simulink model "bench"  (R2025b)
settings: Solver=ode4  StartTime=0.0  StopTime=inf  FixedStep=Ts_gcs  RelTol=1e-3
InitFcn:
  | bench_init_fcn(mocap);
undefined symbols (not defined in the file): mocap, Ts_gcs
libraries: instrumentseriallib x2, sldrtlib x1
settings Model: DataDictionary=project.sldd  SimulationMode=accelerator  Creator=Nick  LastModifiedBy=Rakete
settings SolverCC: AutoInsertRateTranBlk=on

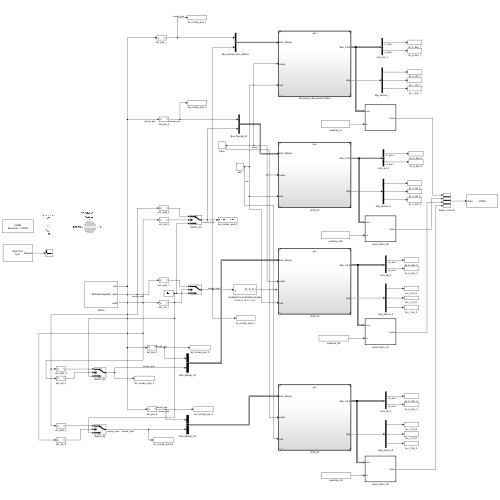
[thumbnail: Simulink's stored preview of the top-level diagram]
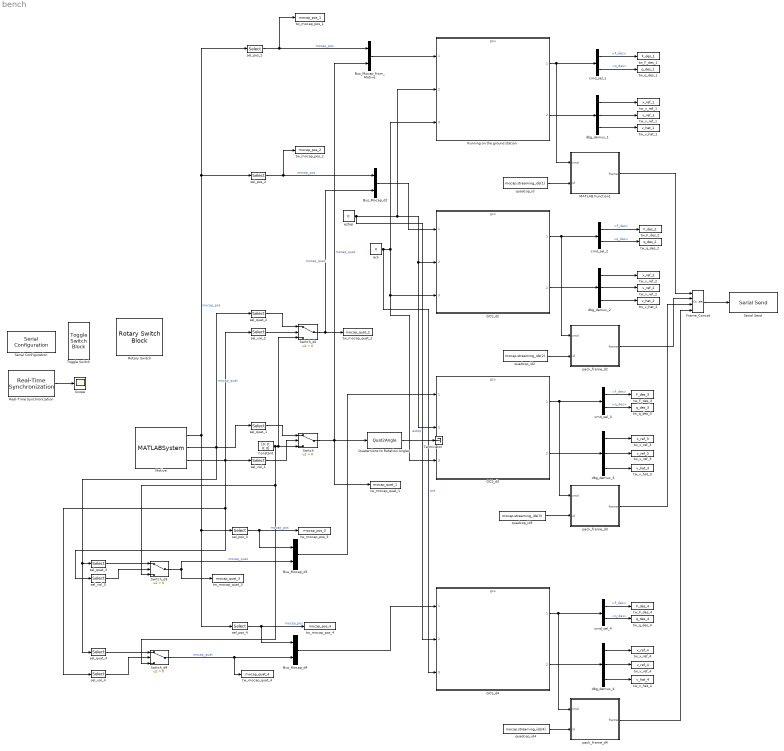
== system bench ==
  Bus_Mocap_d2 : BusCreator  Inputs=2  OutDataTypeStr=Bus: Bus_Mocap
  Bus_Mocap_d3 : BusCreator  Inputs=2  OutDataTypeStr=Bus: Bus_Mocap
  Bus_Mocap_d4 : BusCreator  Inputs=2  OutDataTypeStr=Bus: Bus_Mocap
  Bus_Mocap_from_Motive : BusCreator  Inputs=2  OutDataTypeStr=Bus: Bus_Mocap
  Constant : Constant  Value=[0; 0; 0; 0]
  Frame_Concat : Concatenate  NumInputs=4
  GCS_d2 : ModelReference  ModelNameDialog=gcu.slx  UsingDefaultArgumentValue=0,0,0  SimulationMode=Normal  ModelReferenceVersion=1.334
  GCS_d3 : ModelReference  ModelNameDialog=gcu.slx  UsingDefaultArgumentValue=0,0,0  SimulationMode=Normal  ModelReferenceVersion=1.334
  GCS_d4 : ModelReference  ModelNameDialog=gcu.slx  UsingDefaultArgumentValue=0,0,0  SimulationMode=Normal  ModelReferenceVersion=1.334
  MATLAB Function1 : MATLAB Function  TreatAsAtomicUnit=on
  Motive : MATLABSystem  System=MotiveMocapMulti  HostIP=mocap.host_ip  ClientIP=mocap.client_ip  StreamingIDs=mocap.streaming_ids  SampleTimeSec=Ts_gcs  Verbose=on
      mask Type: MotiveMocapMulti
  Quaternions to Rotation Angles : Quat2Angle
      settings: AttributesFormatString=Rotation Order: %<rotationOrder>
  Real-Time Synchronization : sldrtlib/Real-Time Synchronization  SampleTime=Ts_gcs  MaxMissedTicks=inf  ShowMissedTicks=on  YieldWhenWaiting=off
  Rotary Switch : RotarySwitchBlock
  Running on the ground station : ModelReference  ModelNameDialog=gcu.slx  UsingDefaultArgumentValue=0,0,0  SimulationMode=Normal  ModelReferenceVersion=1.334
  Scope : Scope
      settings: ActiveDisplayYMinimum=-1  ActiveDisplayYMaximum=1
  Serial Configuration : instrumentseriallib/Serial Configuration  Priority=-200000  PortSel=COM4  Port=COM4  ComPort=COM4  BaudRate=115200  DataBits=8  Parity=none  StopBits=1  ByteOrder=little-endian  FlowControl=none  Timeout=10  SimulateUsing=Interpreted execution  BlockInModel=on  aMode=1
      settings: LibrarySourceBlock=c2000lib/Host Communication/Serial Configuration
  Serial Send : instrumentseriallib/Serial Send  Priority=1  PortSel=COM4  Port=COM4  ComPort=COM4  Header=[]  Terminator=<none>  CustomTerminator=[]  EnableBlockingMode=on  SimulateUsing=Interpreted execution  BlockInModel=on  aMode=1
      settings: LibrarySourceBlock=c2000lib/Host Communication/Serial Send
  Switch : Switch  Criteria=u2 > Threshold  SaturateOnIntegerOverflow=off  InputSameDT=off
  Switch_d2 : Switch  Criteria=u2 > Threshold  SaturateOnIntegerOverflow=off  InputSameDT=off
  Switch_d3 : Switch  Criteria=u2 > Threshold  SaturateOnIntegerOverflow=off  InputSameDT=off
  Switch_d4 : Switch  Criteria=u2 > Threshold  SaturateOnIntegerOverflow=off  InputSameDT=off
  Terminator : Terminator
  Toggle Switch : ToggleSwitchBlock
  ack : Constant  Value=0  OutDataTypeStr=boolean
  cmd_sel_{1..4} (4 alike) : BusSelector  OutputSignals=F_des,q_des
  dbg_demux_{1..4} (4 alike) : Demux  Outputs=[3 3 3]
  estop : Constant  Value=0  OutDataTypeStr=uint8
  pack_frame_d2 : MATLAB Function  TreatAsAtomicUnit=on
  pack_frame_d3 : MATLAB Function  TreatAsAtomicUnit=on
  pack_frame_d4 : MATLAB Function  TreatAsAtomicUnit=on
  quadcop_id : Constant  Value=mocap.streaming_ids(1)  OutDataTypeStr=uint8
  quadcop_id2 : Constant  Value=mocap.streaming_ids(2)  OutDataTypeStr=uint8
  quadcop_id3 : Constant  Value=mocap.streaming_ids(3)  OutDataTypeStr=uint8
  quadcop_id4 : Constant  Value=mocap.streaming_ids(4)  OutDataTypeStr=uint8
  sel_pos_1 : Selector  NumberOfDimensions=2  IndexOptions=Select all,Index vector (dialog)  Indices=1,1  OutputSizes=1
  sel_pos_2 : Selector  NumberOfDimensions=2  IndexOptions=Select all,Index vector (dialog)  Indices=1,2  OutputSizes=1
  sel_pos_3 : Selector  NumberOfDimensions=2  IndexOptions=Select all,Index vector (dialog)  Indices=1,3  OutputSizes=1
  sel_pos_4 : Selector  NumberOfDimensions=2  IndexOptions=Select all,Index vector (dialog)  Indices=1,4  OutputSizes=1
  sel_quat_1 : Selector  NumberOfDimensions=2  IndexOptions=Select all,Index vector (dialog)  Indices=1,1  OutputSizes=1
  sel_quat_2 : Selector  NumberOfDimensions=2  IndexOptions=Select all,Index vector (dialog)  Indices=1,2  OutputSizes=1
  sel_quat_3 : Selector  NumberOfDimensions=2  IndexOptions=Select all,Index vector (dialog)  Indices=1,3  OutputSizes=1
  sel_quat_4 : Selector  NumberOfDimensions=2  IndexOptions=Select all,Index vector (dialog)  Indices=1,4  OutputSizes=1
  sel_val_1 : Selector  IndexOptions=Index vector (dialog)  Indices=1  OutputSizes=1
  sel_val_2 : Selector  IndexOptions=Index vector (dialog)  Indices=2  OutputSizes=1
  sel_val_3 : Selector  IndexOptions=Index vector (dialog)  Indices=3  OutputSizes=1
  sel_val_4 : Selector  IndexOptions=Index vector (dialog)  Indices=4  OutputSizes=1
  tw_F_des_1 : ToWorkspace  VariableName=F_des_1  SaveFormat=Timeseries  SampleTime=Ts_gcs
  tw_F_des_2 : ToWorkspace  VariableName=F_des_2  SaveFormat=Timeseries  SampleTime=Ts_gcs
  tw_F_des_3 : ToWorkspace  VariableName=F_des_3  SaveFormat=Timeseries  SampleTime=Ts_gcs
  tw_F_des_4 : ToWorkspace  VariableName=F_des_4  SaveFormat=Timeseries  SampleTime=Ts_gcs
  tw_mocap_pos_1 : ToWorkspace  VariableName=mocap_pos_1  SaveFormat=Timeseries  SampleTime=Ts_gcs
  tw_mocap_pos_2 : ToWorkspace  VariableName=mocap_pos_2  SaveFormat=Timeseries  SampleTime=Ts_gcs
  tw_mocap_pos_3 : ToWorkspace  VariableName=mocap_pos_3  SaveFormat=Timeseries  SampleTime=Ts_gcs
  tw_mocap_pos_4 : ToWorkspace  VariableName=mocap_pos_4  SaveFormat=Timeseries  SampleTime=Ts_gcs
  tw_mocap_quat_1 : ToWorkspace  VariableName=mocap_quat_1  SaveFormat=Timeseries  SampleTime=Ts_gcs
  tw_mocap_quat_2 : ToWorkspace  VariableName=mocap_quat_2  SaveFormat=Timeseries  SampleTime=Ts_gcs
  tw_mocap_quat_3 : ToWorkspace  VariableName=mocap_quat_3  SaveFormat=Timeseries  SampleTime=Ts_gcs
  tw_mocap_quat_4 : ToWorkspace  VariableName=mocap_quat_4  SaveFormat=Timeseries  SampleTime=Ts_gcs
  tw_q_des_1 : ToWorkspace  VariableName=q_des_1  SaveFormat=Timeseries  SampleTime=Ts_gcs
  tw_q_des_2 : ToWorkspace  VariableName=q_des_2  SaveFormat=Timeseries  SampleTime=Ts_gcs
  tw_q_des_3 : ToWorkspace  VariableName=q_des_3  SaveFormat=Timeseries  SampleTime=Ts_gcs
  tw_q_des_4 : ToWorkspace  VariableName=q_des_4  SaveFormat=Timeseries  SampleTime=Ts_gcs
  tw_v_hat_1 : ToWorkspace  VariableName=v_hat_1  SaveFormat=Timeseries  SampleTime=Ts_gcs
  tw_v_hat_2 : ToWorkspace  VariableName=v_hat_2  SaveFormat=Timeseries  SampleTime=Ts_gcs
  tw_v_hat_3 : ToWorkspace  VariableName=v_hat_3  SaveFormat=Timeseries  SampleTime=Ts_gcs
  tw_v_hat_4 : ToWorkspace  VariableName=v_hat_4  SaveFormat=Timeseries  SampleTime=Ts_gcs
  tw_v_ref_1 : ToWorkspace  VariableName=v_ref_1  SaveFormat=Timeseries  SampleTime=Ts_gcs
  tw_v_ref_2 : ToWorkspace  VariableName=v_ref_2  SaveFormat=Timeseries  SampleTime=Ts_gcs
  tw_v_ref_3 : ToWorkspace  VariableName=v_ref_3  SaveFormat=Timeseries  SampleTime=Ts_gcs
  tw_v_ref_4 : ToWorkspace  VariableName=v_ref_4  SaveFormat=Timeseries  SampleTime=Ts_gcs
  tw_x_ref_1 : ToWorkspace  VariableName=x_ref_1  SaveFormat=Timeseries  SampleTime=Ts_gcs
  tw_x_ref_2 : ToWorkspace  VariableName=x_ref_2  SaveFormat=Timeseries  SampleTime=Ts_gcs
  tw_x_ref_3 : ToWorkspace  VariableName=x_ref_3  SaveFormat=Timeseries  SampleTime=Ts_gcs
  tw_x_ref_4 : ToWorkspace  VariableName=x_ref_4  SaveFormat=Timeseries  SampleTime=Ts_gcs
  wires:
  sel_val_1/1 -> Switch/2
  Motive/3 -> sel_val_3/1, sel_val_4/1, sel_val_1/1, sel_val_2/1
  Motive/1 -> sel_pos_3/1, sel_pos_4/1, sel_pos_2/1, sel_pos_1/1  "mocap_pos"
  Motive/2 -> sel_quat_3/1, sel_quat_4/1, sel_quat_1/1, sel_quat_2/1  "mocap_quat"
  quadcop_id2/1 -> pack_frame_d2/2(id)
  Real-Time Synchronization/1 -> Scope/1
  dbg_demux_2/1 -> tw_x_ref_2/1
  sel_pos_1/1 -> tw_mocap_pos_1/1, Bus_Mocap_from_Motive/1  "mocap_pos"
  sel_val_2/1 -> Switch_d2/2
  Switch_d2/1 -> tw_mocap_quat_2/1, Bus_Mocap_d2/2  "mocap_quat"
  sel_quat_1/1 -> Switch/1
  sel_quat_2/1 -> Switch_d2/1
  sel_pos_2/1 -> Bus_Mocap_d2/1, tw_mocap_pos_2/1  "mocap_pos"
  Constant/1 -> Switch_d3/3, Switch_d4/3, Switch/3, Switch_d2/3
  GCS_d2/1 -> pack_frame_d2/1(cmd), cmd_sel_2/1
  Switch/1 -> Quaternions to Rotation Angles/1, tw_mocap_quat_1/1, Bus_Mocap_from_Motive/2  "mocap_quat"
  Running on the ground station/2 -> dbg_demux_1/1
  Bus_Mocap_from_Motive/1 -> Running on the ground station/1
  MATLAB Function1/1(frame) -> Frame_Concat/1
  Bus_Mocap_d2/1 -> GCS_d2/1
  dbg_demux_1/2 -> tw_v_ref_1/1
  estop/1 -> GCS_d3/2, GCS_d2/2, Running on the ground station/2, GCS_d4/2  "estop"
  ack/1 -> GCS_d3/3, GCS_d2/3, Running on the ground station/3, GCS_d4/3  "ack"
  dbg_demux_1/3 -> tw_v_hat_1/1
  Running on the ground station/1 -> MATLAB Function1/1(cmd), cmd_sel_1/1
  Quaternions to Rotation Angles/1 -> Terminator/1
  GCS_d2/2 -> dbg_demux_2/1
  quadcop_id/1 -> MATLAB Function1/2(id)
  cmd_sel_1/1 -> tw_F_des_1/1  "<F_des>"
  cmd_sel_1/2 -> tw_q_des_1/1  "<q_des>"
  dbg_demux_1/1 -> tw_x_ref_1/1
  cmd_sel_2/1 -> tw_F_des_2/1  "<F_des>"
  cmd_sel_2/2 -> tw_q_des_2/1  "<q_des>"
  dbg_demux_2/2 -> tw_v_ref_2/1
  dbg_demux_2/3 -> tw_v_hat_2/1
  pack_frame_d2/1(frame) -> Frame_Concat/2
  Frame_Concat/1 -> Serial Send/1
  sel_pos_3/1 -> Bus_Mocap_d3/1, tw_mocap_pos_3/1  "mocap_pos"
  sel_quat_3/1 -> Switch_d3/1
  sel_val_3/1 -> Switch_d3/2
  Switch_d3/1 -> Bus_Mocap_d3/2, tw_mocap_quat_3/1  "mocap_quat"
  Bus_Mocap_d3/1 -> GCS_d3/1
  GCS_d3/1 -> pack_frame_d3/1(cmd), cmd_sel_3/1
  quadcop_id3/1 -> pack_frame_d3/2(id)
  pack_frame_d3/1(frame) -> Frame_Concat/3
  GCS_d3/2 -> dbg_demux_3/1
  dbg_demux_3/1 -> tw_x_ref_3/1
  dbg_demux_3/2 -> tw_v_ref_3/1
  dbg_demux_3/3 -> tw_v_hat_3/1
  cmd_sel_3/1 -> tw_F_des_3/1  "<F_des>"
  cmd_sel_3/2 -> tw_q_des_3/1  "<q_des>"
  sel_quat_4/1 -> Switch_d4/1
  sel_val_4/1 -> Switch_d4/2
  sel_pos_4/1 -> Bus_Mocap_d4/1, tw_mocap_pos_4/1  "mocap_pos"
  Switch_d4/1 -> tw_mocap_quat_4/1, Bus_Mocap_d4/2  "mocap_quat"
  Bus_Mocap_d4/1 -> GCS_d4/1
  GCS_d4/1 -> pack_frame_d4/1(cmd), cmd_sel_4/1
  GCS_d4/2 -> dbg_demux_4/1
  quadcop_id4/1 -> pack_frame_d4/2(id)
  pack_frame_d4/1(frame) -> Frame_Concat/4
  cmd_sel_4/1 -> tw_F_des_4/1  "<F_des>"
  cmd_sel_4/2 -> tw_q_des_4/1  "<q_des>"
  dbg_demux_4/1 -> tw_x_ref_4/1
  dbg_demux_4/2 -> tw_v_ref_4/1
  dbg_demux_4/3 -> tw_v_hat_4/1

== matlab function bench/pack_frame_d2 ==
  data: cmd input Bus: Bus_Cmd; frame output uint8 size=[1 82]; id input uint8 size=[1 1]
function frame = pack_gcs_frame_sl(cmd, id)
%#codegen
% WRAPPER — haelt KEINE Logik. Single Source of Truth ist
% scripts\functions\pack_gcs_frame.m; dieser Block ruft sie nur auf.
% Grund: .slx ist binaer -> Inline-Kopien driften unbemerkt und sind im
% git-Diff unsichtbar (Session 9: 2 von 11 Bloecken waren abgewichen).
% Name MUSS abweichen (_sl), sonst schattet er die externe Funktion.
frame = pack_gcs_frame(cmd, id);
end

== matlab function bench/pack_frame_d3 ==
  data: cmd input Bus: Bus_Cmd; frame output uint8 size=[1 82]; id input uint8 size=[1 1]
function frame = pack_gcs_frame_sl(cmd, id)
%#codegen
% WRAPPER — haelt KEINE Logik. Single Source of Truth ist
% scripts\functions\pack_gcs_frame.m; dieser Block ruft sie nur auf.
% Grund: .slx ist binaer -> Inline-Kopien driften unbemerkt und sind im
% git-Diff unsichtbar (Session 9: 2 von 11 Bloecken waren abgewichen).
% Name MUSS abweichen (_sl), sonst schattet er die externe Funktion.
frame = pack_gcs_frame(cmd, id);
end

== matlab function bench/pack_frame_d4 ==
  data: cmd input Bus: Bus_Cmd; frame output uint8 size=[1 82]; id input uint8 size=[1 1]
function frame = pack_gcs_frame_sl(cmd, id)
%#codegen
% WRAPPER — haelt KEINE Logik. Single Source of Truth ist
% scripts\functions\pack_gcs_frame.m; dieser Block ruft sie nur auf.
% Grund: .slx ist binaer -> Inline-Kopien driften unbemerkt und sind im
% git-Diff unsichtbar (Session 9: 2 von 11 Bloecken waren abgewichen).
% Name MUSS abweichen (_sl), sonst schattet er die externe Funktion.
frame = pack_gcs_frame(cmd, id);
end

== matlab function bench/MATLAB Function1 ==
  data: cmd input Bus: Bus_Cmd; frame output uint8 size=[1 82]; id input uint8 size=[1 1]
function frame = pack_gcs_frame_sl(cmd, id)
%#codegen
% WRAPPER — haelt KEINE Logik. Single Source of Truth ist
% scripts\functions\pack_gcs_frame.m; dieser Block ruft sie nur auf.
% Grund: .slx ist binaer -> Inline-Kopien driften unbemerkt und sind im
% git-Diff unsichtbar (Session 9: 2 von 11 Bloecken waren abgewichen).
% Name MUSS abweichen (_sl), sonst schattet er die externe Funktion.
frame = pack_gcs_frame(cmd, id);
end
